simulink model "Linm_MSP"  (Simulink 7.5)
settings: Solver=ode3  StartTime=0.0  StopTime=10.0  FixedStep=0.02  RelTol=1e-3
undefined symbols (not defined in the file or in its folder): Adr, Bdr, Cdr, Ddr, q1, q2, q3, q4
settings Model: Creator=fclaveau  LastModifiedBy=fclaveau  BufferReuse=off
settings OptimizationCC: InlineParams=on  BufferReuse=off

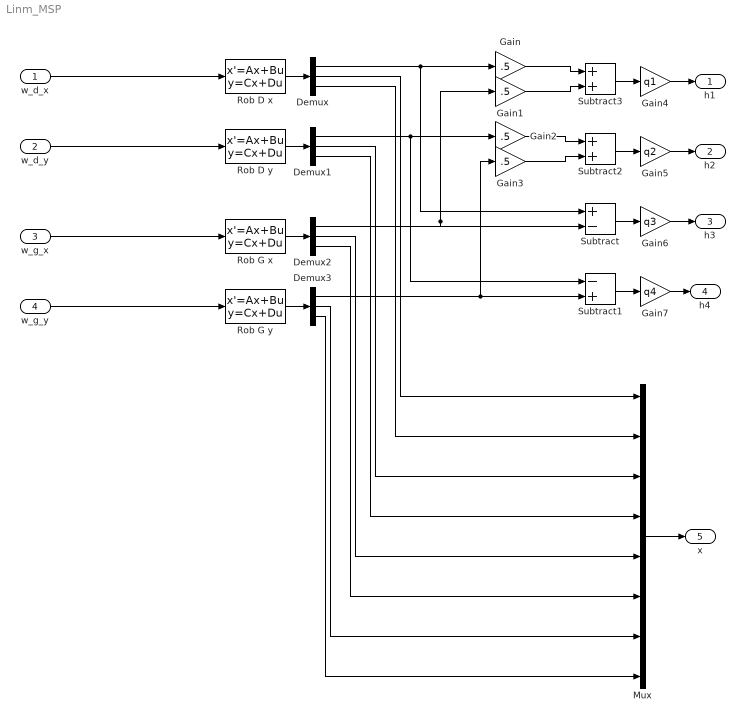
== system Linm_MSP ==
  w_d_x : Inport  OutDataType=fixdt(1, 16)  OutScaling=2^0
  w_d_y : Inport  Port=2  OutDataType=fixdt(1, 16)  OutScaling=2^0
  w_g_x : Inport  Port=3  OutDataType=fixdt(1, 16)  OutScaling=2^0
  w_g_y : Inport  Port=4  OutDataType=fixdt(1, 16)  OutScaling=2^0
  Demux{,1..3} (4 alike) : Demux  Outputs=3
  Gain{,1..3} (4 alike) : Gain  Gain=.5  ParameterDataType=fixdt(1, 16)  ParameterScaling=2^0  OutDataType=fixdt(1, 16)  OutScaling=2^0
  Gain4 : Gain  Gain=q1  ParameterDataType=fixdt(1, 16)  ParameterScaling=2^0  OutDataType=fixdt(1, 16)  OutScaling=2^0
  Gain5 : Gain  Gain=q2  ParameterDataType=fixdt(1, 16)  ParameterScaling=2^0  OutDataType=fixdt(1, 16)  OutScaling=2^0
  Gain6 : Gain  Gain=q3  ParameterDataType=fixdt(1, 16)  ParameterScaling=2^0  OutDataType=fixdt(1, 16)  OutScaling=2^0
  Gain7 : Gain  Gain=q4  ParameterDataType=fixdt(1, 16)  ParameterScaling=2^0  OutDataType=fixdt(1, 16)  OutScaling=2^0
  Mux : Mux  Inputs=8
  "Rob D x " : StateSpace  A=Adr  B=Bdr  C=Cdr  D=Ddr
  Rob D y : StateSpace  A=Adr  B=Bdr  C=Cdr  D=Ddr
  Rob G x : StateSpace  A=Adr  B=Bdr  C=Cdr  D=Ddr
  Rob G y : StateSpace  A=Adr  B=Bdr  C=Cdr  D=Ddr
  Subtract : Sum  Inputs=+-  OutDataType=fixdt(1, 16)  OutScaling=2^-10
  Subtract1 : Sum  Inputs=-+  OutDataType=fixdt(1, 16)  OutScaling=2^-10
  Subtract2 : Sum  OutDataType=fixdt(1, 16)  OutScaling=2^-10
  Subtract3 : Sum  OutDataType=fixdt(1, 16)  OutScaling=2^-10
  h1 : Outport  OutDataType=fixdt(1, 16)  OutScaling=2^0
  h2 : Outport  Port=2  OutDataType=fixdt(1, 16)  OutScaling=2^0
  h3 : Outport  Port=3  OutDataType=fixdt(1, 16)  OutScaling=2^0
  h4 : Outport  Port=4  OutDataType=fixdt(1, 16)  OutScaling=2^0
  x : Outport  Port=5  OutDataType=fixdt(1, 16)  OutScaling=2^0
  wires:
  Gain/1 -> Subtract3/1
  Gain1/1 -> Subtract3/2
  "Rob D x "/1 -> Demux/1
  Rob D y/1 -> Demux1/1
  Rob G x/1 -> Demux2/1
  Rob G y/1 -> Demux3/1
  Demux/1 -> Gain/1, Subtract/1
  Demux2/1 -> Gain1/1, Subtract/2
  Gain2/1 -> Subtract2/1
  Gain3/1 -> Subtract2/2
  Demux1/1 -> Gain2/1, Subtract1/1
  Demux3/1 -> Gain3/1, Subtract1/2
  Subtract3/1 -> Gain4/1
  Subtract2/1 -> Gain5/1
  Subtract/1 -> Gain6/1
  Subtract1/1 -> Gain7/1
  Demux/2 -> Mux/1
  Demux/3 -> Mux/2
  Demux1/2 -> Mux/3
  Demux1/3 -> Mux/4
  Demux2/2 -> Mux/5
  Demux2/3 -> Mux/6
  Demux3/2 -> Mux/7
  Demux3/3 -> Mux/8
  Gain4/1 -> h1/1
  Gain5/1 -> h2/1
  Gain6/1 -> h3/1
  Gain7/1 -> h4/1
  Mux/1 -> x/1
  w_d_x/1 -> "Rob D x "/1
  w_d_y/1 -> Rob D y/1
  w_g_x/1 -> Rob G x/1
  w_g_y/1 -> Rob G y/1
